simulink model "q5"  (R2016a)
settings: Solver=VariableStepAuto  StartTime=0.0  StopTime=10000  MaxStep=0.01  RelTol=1e-4
settings Model: Creator=derakhshani4476  LastModifiedBy=derakhshani4476
settings DataIOCC: LimitDataPoints=on  SaveOutput=off  SaveTime=off
settings OptimizationCC: ExpressionDepthLimit=2147483647  LifeSpan=1
settings DebuggingCC: UnderspecifiedInitializationDetection=Classic  MergeDetectMultiDrivingBlocksExec=none  FcnCallInpInsideContextMsg=EnableAllAsWarning  AllowSymbolicDim=off  StateNameClashWarn=warning
settings GRTTargetCC: CombineOutputUpdateFcns=off  GRTInterface=on

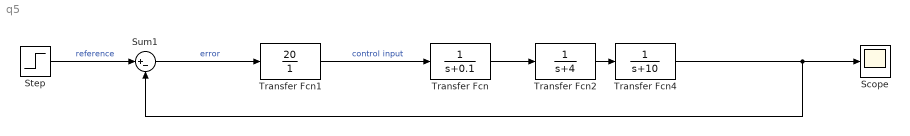
== system q5 ==
  Scope : Scope
  Step : Step  Time=0  After=100  SampleTime=0
  Sum1 : Sum  Inputs=|+-
  Transfer Fcn : TransferFcn  Denominator="[ 1 0.1  ]"
  Transfer Fcn1 : TransferFcn  Numerator=[20]  Denominator="[ 0 1  ]"
  Transfer Fcn2 : TransferFcn  Denominator="[ 1 4  ]"
  Transfer Fcn4 : TransferFcn  Denominator="[ 1 10  ]"
  wires:
  Step/1 -> Sum1/1  "reference"
  Sum1/1 -> Transfer Fcn1/1  "error"
  Transfer Fcn/1 -> Transfer Fcn2/1
  Transfer Fcn2/1 -> Transfer Fcn4/1
  Transfer Fcn4/1 -> Sum1/2, Scope/1
  Transfer Fcn1/1 -> Transfer Fcn/1  "control input"
